simulink library "lfc"  (Simulink 8.2)
settings: Solver=ode1  StartTime=0.0  StopTime=Inf  FixedStep=0.001  RelTol=1e-3
PostLoadFcn:
  | , if any(exist('dsrtsu_mdlpostloadfcn', 'file') == [2, 3, 6]), try dsrtsu_mdlpostloadfcn('Execute', bdroot); catch fprintf('Error in PostLoadFcn (dsrtsu_mdlpostloadfcn) for model "%s":\n %s\n', bdroot, lasterr); end, end,
undefined symbols (not defined in the file or in its folder): ALFC_CenterC0_m, ALFC_ErrorY_m, ALFC_VehSpd_X_kph, C_TASK_5MS_S, C_TICK_TIME_S, ENUM_LFCSTATE_ADASFAILURE, ENUM_LFCSTATE_AUTOSTEERING, ENUM_LFCSTATE_DEGRADED, ENUM_LFCSTATE_DISABLED, ENUM_LFCSTATE_EPSRECOVERYPENDING, ENUM_LFCSTATE_OFF, ENUM_LFCSTATE_SOFTEN, ENUM_LFCSTATE_STANDBY, FALSE, KAPP_StrCenterOffset_deg, KAPP_Wheel2SteerRatio_rat, KAPP_WheelBase_m, KLFC_DDecRate_m, KLFC_DIncRate_m, KLFC_IGainLowerLimit_rad, KLFC_IGainUpperLimit_rad, MLFC_C0ErrorDist_m, MLFC_ControlGain_rat, MLFC_KgainRatio_rat, MLFC_KusCoeff_rat, MLFC_LookAheadDistGain_rat, TRUE
libraries: hcu_lib x7, simulink x2
settings Model: DSRTSU_INTERNAL_RTI_VER=450  DSRTSU_INTERNAL_RTI_TYPE=rti1401  RTICANMMDATA=struct('GeneralSetupData',struct('modelroot','C:\ADAS\trunk\ADAS_Softwares\HTDragon\software\sw_development\arch\app\lfc','generalsettings',struct('filesettings',struct('destfolder',struct('Name','RTICANMM_FILES','Check',1),'buildfolder',struct('Name','.','Check',1),'AbsDestfolder',struct('Name','C:\ADAS\trunk\ADAS_Softwares\HTDragon\software\sw_development\arch\app\lfc\RTICANMM_FILES'),'AbsBuildfolder',struct('Name','C:\ADAS\trunk\ADAS_Softwares\HTDragon\software\sw_development\arch\app\lfc'))),'options',struct('addpaths',1,'rmpaths',1,'addtrcexclusion',logical(1),'cannavigator',struct('checkmonitoring',0),'show_usrtrc',0,'use_usrtrc',0),'advanced',struct('options',[1 1 1 1 1 1 1 1 1 1 1 1 1 1 1 1 1 1 1 1 1 1 1 1 1 1 1 1 1 1 1 1 1 1 1 1 1 1 1 1 1 1 1 1 1 1 1 1 1 1 1 1 1 1 1 1 1 1 1 1 1 1 1 1 1 1 1 1 1 1 1 1 1 1 1 1 1 1 1 1 1 1 1 1 1 1 1 1 1 1 1 1 1 1 1 1 1 1 1 1]),'MPSetup',{{}},'modelname','lfc','block','lfc'))  DSRTSU_INTERNAL_RTIFPGA=40  Creator=14014  LastModifiedBy=13192

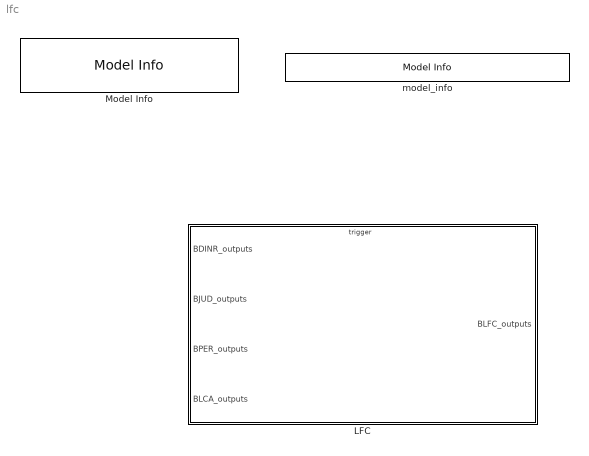
== system lfc ==
  LFC : Subsystem
  Model Info : simulink/Model-Wide Utilities/Model Info  InitialBlockCM=None  BlockCM=None  Frame=on  DisplayStringWithTags=|  HorizontalTextAlignment=Left  LeftAlignmentValue=0.02  SourceBlockDiagram=lfc  TagMaxNumber=20
      | Model Version        : %<ModelVersion>
      | Creator                   : %<Creator>
      | Last Modified by    : %<LastModifiedBy>
  model_info : simulink/Model-Wide Utilities/Model Info  InitialBlockCM=None  BlockCM=None  Frame=on  DisplayStringWithTags=$Id: lfc.mdl 1621 2017-09-19 03:18:21Z bcluan $  HorizontalTextAlignment=Center  LeftAlignmentValue=0.5  SourceBlockDiagram=lfc  TagMaxNumber=20

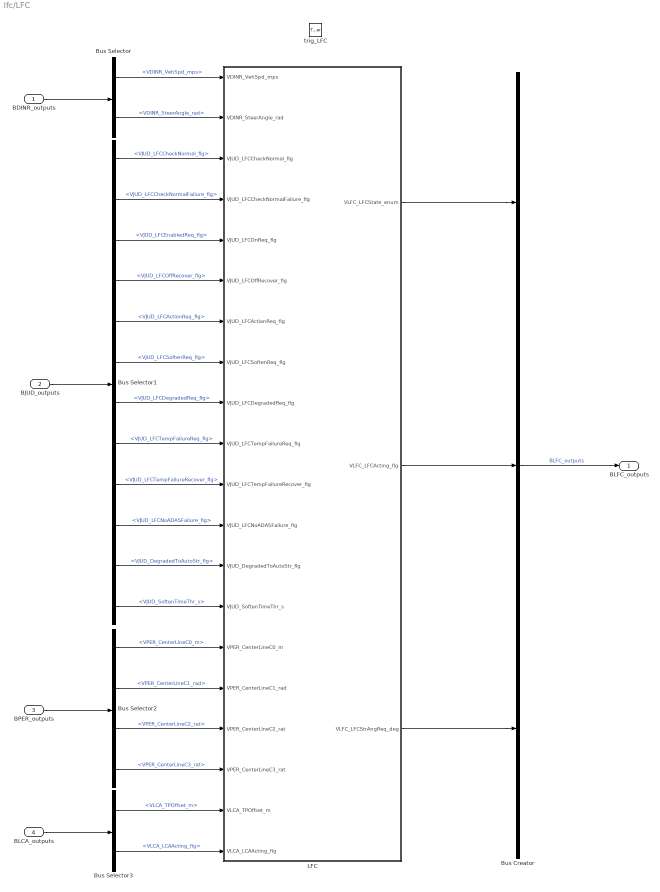
== system lfc/LFC ==
  BDINR_outputs : Inport  OutDataTypeStr=Bus: BDINR_outputs
  BJUD_outputs : Inport  Port=2  OutDataTypeStr=Bus: BJUD_outputs
  BPER_outputs : Inport  Port=3  OutDataTypeStr=Bus: BPER_outputs
  BLCA_outputs : Inport  Port=4  OutDataTypeStr=Bus: BLCA_outputs
  trig_LFC : TriggerPort  TriggerType=function-call
      settings: AttributesFormatString=State = %<StatesWhenEnabling>
  Bus Creator : BusCreator  Inputs=3  OutDataTypeStr=Bus: BLFC_outputs
  Bus Selector : BusSelector  OutputSignals=VDINR_VehSpd_mps,VDINR_SteerAngle_rad
  Bus Selector1 : BusSelector  OutputSignals=VJUD_LFCCheckNormal_flg,VJUD_LFCCheckNormalFailure_flg,VJUD_LFCEnabledReq_flg,VJUD_LFCOffRecover_flg,VJUD_LFCActionReq_flg,VJUD_LFCSoftenReq_flg,VJUD_LFCDegradedReq_flg,VJUD_LFCTempFailureReq_flg,VJUD_LFCTempFailureRecover_flg,VJUD_LFCNoADASFailure_flg,VJUD_DegradedToAutoStr_flg,VJUD_SoftenTimeThr_s
  Bus Selector2 : BusSelector  OutputSignals=VPER_CenterLineC0_m,VPER_CenterLineC1_rad,VPER_CenterLineC2_rat,VPER_CenterLineC3_rat
  Bus Selector3 : BusSelector  OutputSignals=VLCA_TPOffset_m,VLCA_LCAActing_flg
  LFC : Subsystem
  BLFC_outputs : Outport  OutDataTypeStr=Bus: BLFC_outputs
  wires:
  Bus Creator/1 -> BLFC_outputs/1  "BLFC_outputs"
  BDINR_outputs/1 -> Bus Selector/1
  BPER_outputs/1 -> Bus Selector2/1
  LFC/3(VLFC_LFCStrAngReq_deg) -> Bus Creator/3
  LFC/2(VLFC_LFCActing_flg) -> Bus Creator/2
  LFC/1(VLFC_LFCState_enum) -> Bus Creator/1
  BJUD_outputs/1 -> Bus Selector1/1
  Bus Selector/1 -> LFC/1(VDINR_VehSpd_mps)  "<VDINR_VehSpd_mps>"
  Bus Selector/2 -> LFC/2(VDINR_SteerAngle_rad)  "<VDINR_SteerAngle_rad>"
  Bus Selector1/1 -> LFC/3(VJUD_LFCCheckNormal_flg)  "<VJUD_LFCCheckNormal_flg>"
  Bus Selector1/3 -> LFC/5(VJUD_LFCOnReq_flg)  "<VJUD_LFCEnabledReq_flg>"
  Bus Selector1/4 -> LFC/6(VJUD_LFCOffRecover_flg)  "<VJUD_LFCOffRecover_flg>"
  Bus Selector1/5 -> LFC/7(VJUD_LFCActionReq_flg)  "<VJUD_LFCActionReq_flg>"
  Bus Selector1/6 -> LFC/8(VJUD_LFCSoftenReq_flg)  "<VJUD_LFCSoftenReq_flg>"
  Bus Selector1/7 -> LFC/9(VJUD_LFCDegradedReq_flg)  "<VJUD_LFCDegradedReq_flg>"
  Bus Selector1/8 -> LFC/10(VJUD_LFCTempFailureReq_flg)  "<VJUD_LFCTempFailureReq_flg>"
  Bus Selector1/9 -> LFC/11(VJUD_LFCTempFailureRecover_flg)  "<VJUD_LFCTempFailureRecover_flg>"
  Bus Selector1/10 -> LFC/12(VJUD_LFCNoADASFailure_flg)  "<VJUD_LFCNoADASFailure_flg>"
  Bus Selector1/11 -> LFC/13(VJUD_DegradedToAutoStr_flg)  "<VJUD_DegradedToAutoStr_flg>"
  BLCA_outputs/1 -> Bus Selector3/1
  Bus Selector1/12 -> LFC/14(VJUD_SoftenTimeThr_s)  "<VJUD_SoftenTimeThr_s>"
  Bus Selector2/4 -> LFC/18(VPER_CenterLineC3_rat)  "<VPER_CenterLineC3_rat>"
  Bus Selector2/2 -> LFC/16(VPER_CenterLineC1_rad)  "<VPER_CenterLineC1_rad>"
  Bus Selector2/1 -> LFC/15(VPER_CenterLineC0_m)  "<VPER_CenterLineC0_m>"
  Bus Selector2/3 -> LFC/17(VPER_CenterLineC2_rat)  "<VPER_CenterLineC2_rat>"
  Bus Selector3/1 -> LFC/19(VLCA_TPOffset_m)  "<VLCA_TPOffset_m>"
  Bus Selector3/2 -> LFC/20(VLCA_LCAActing_flg)  "<VLCA_LCAActing_flg>"
  Bus Selector1/2 -> LFC/4(VJUD_LFCCheckNormalFailure_flg)  "<VJUD_LFCCheckNormalFailure_flg>"

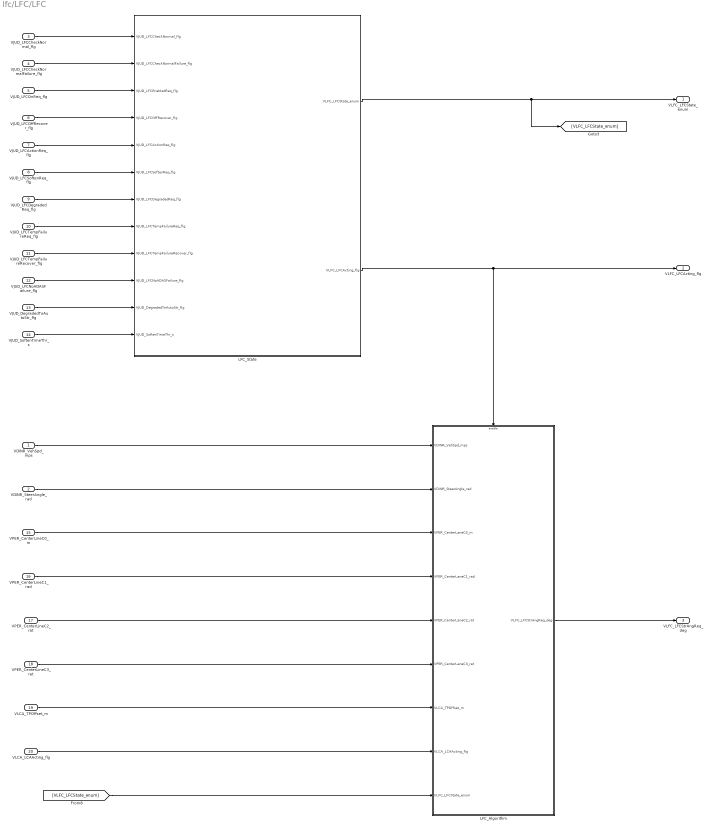
== system lfc/LFC/LFC ==
  VDINR_VehSpd_mps : Inport
  VDINR_SteerAngle_rad : Inport  Port=2
  VJUD_LFCCheckNormal_flg : Inport  Port=3
  VJUD_LFCCheckNormalFailure_flg : Inport  Port=4
  VJUD_LFCOnReq_flg : Inport  Port=5
  VJUD_LFCOffRecover_flg : Inport  Port=6
  VJUD_LFCActionReq_flg : Inport  Port=7
  VJUD_LFCSoftenReq_flg : Inport  Port=8
  VJUD_LFCDegradedReq_flg : Inport  Port=9
  VJUD_LFCTempFailureReq_flg : Inport  Port=10
  VJUD_LFCTempFailureRecover_flg : Inport  Port=11
  VJUD_LFCNoADASFailure_flg : Inport  Port=12
  VJUD_DegradedToAutoStr_flg : Inport  Port=13
  VJUD_SoftenTimeThr_s : Inport  Port=14
  VPER_CenterLineC0_m : Inport  Port=15
  VPER_CenterLineC1_rad : Inport  Port=16
  VPER_CenterLineC2_rat : Inport  Port=17
  VPER_CenterLineC3_rat : Inport  Port=18
  VLCA_TPOffset_m : Inport  Port=19
  VLCA_LCAActing_flg : Inport  Port=20
  LFC_Algorithm : Subsystem  TreatAsAtomicUnit=on
  LFC_State : Stateflow chart  TreatAsAtomicUnit=on
  VLFC_LFCState_enum : Outport  OutputWhenDisabled=reset  InitialOutput=[0]
  VLFC_LFCActing_flg : Outport  Port=2  OutputWhenDisabled=reset  InitialOutput=[0]
  VLFC_LFCStrAngReq_deg : Outport  Port=3  OutputWhenDisabled=reset  InitialOutput=[0]
  wires:
  [VLFC_LFCState_enum] -> LFC_Algorithm/9(VLFC_LFCState_enum)
  VLCA_LCAActing_flg/1 -> LFC_Algorithm/8(VLCA_LCAActing_flg)
  VLCA_TPOffset_m/1 -> LFC_Algorithm/7(VLCA_TPOffset_m)
  VJUD_DegradedToAutoStr_flg/1 -> LFC_State/11(VJUD_DegradedToAutoStr_flg)
  VJUD_LFCNoADASFailure_flg/1 -> LFC_State/10(VJUD_LFCNoADASFailure_flg)
  VJUD_LFCTempFailureRecover_flg/1 -> LFC_State/9(VJUD_LFCTempFailureRecover_flg)
  VJUD_LFCTempFailureReq_flg/1 -> LFC_State/8(VJUD_LFCTempFailureReq_flg)
  VJUD_SoftenTimeThr_s/1 -> LFC_State/12(VJUD_SoftenTimeThr_s)
  LFC_State/1(VLFC_LFCState_enum) -> VLFC_LFCState_enum/1, [VLFC_LFCState_enum]
  LFC_State/2(VLFC_LFCActing_flg) -> VLFC_LFCActing_flg/1, LFC_Algorithm/Enable
  VJUD_LFCDegradedReq_flg/1 -> LFC_State/7(VJUD_LFCDegradedReq_flg)
  VJUD_LFCSoftenReq_flg/1 -> LFC_State/6(VJUD_LFCSoftenReq_flg)
  VJUD_LFCActionReq_flg/1 -> LFC_State/5(VJUD_LFCActionReq_flg)
  VJUD_LFCOffRecover_flg/1 -> LFC_State/4(VJUD_LFCOffRecover_flg)
  VJUD_LFCOnReq_flg/1 -> LFC_State/3(VJUD_LFCEnabledReq_flg)
  VJUD_LFCCheckNormal_flg/1 -> LFC_State/1(VJUD_LFCCheckNormal_flg)
  LFC_Algorithm/1(VLFC_LFCStrAngReq_deg) -> VLFC_LFCStrAngReq_deg/1
  VDINR_SteerAngle_rad/1 -> LFC_Algorithm/2(VDINR_SteerAngle_rad)
  VDINR_VehSpd_mps/1 -> LFC_Algorithm/1(VDINR_VehSpd_mps)
  VPER_CenterLineC0_m/1 -> LFC_Algorithm/3(VPER_CenterLaneC0_m)
  VPER_CenterLineC1_rad/1 -> LFC_Algorithm/4(VPER_CenterLaneC1_rad)
  VPER_CenterLineC2_rat/1 -> LFC_Algorithm/5(VPER_CenterLaneC2_rat)
  VPER_CenterLineC3_rat/1 -> LFC_Algorithm/6(VPER_CenterLaneC3_rat)
  VJUD_LFCCheckNormalFailure_flg/1 -> LFC_State/2(VJUD_LFCCheckNormalFailure_flg)

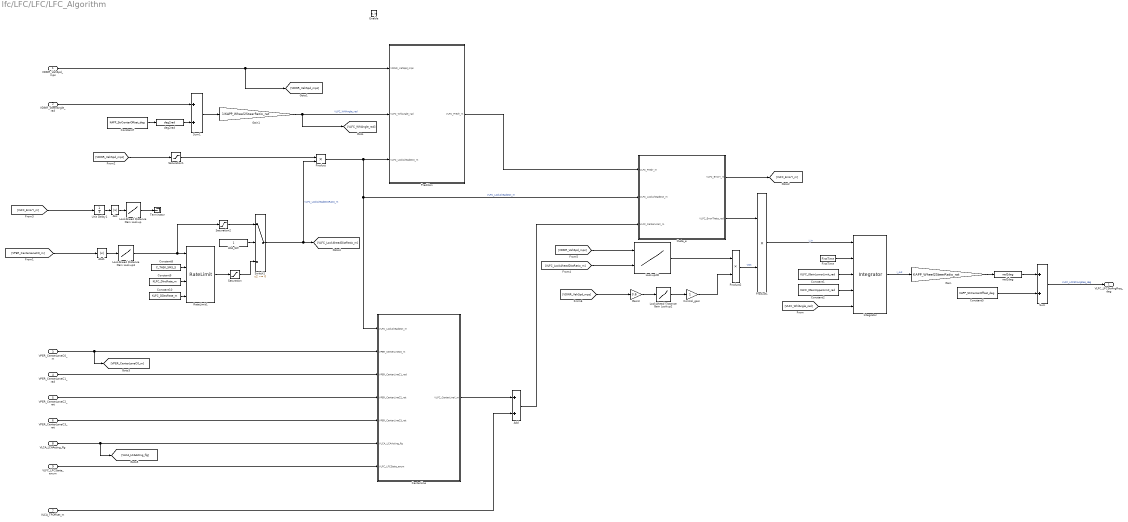
== system lfc/LFC/LFC/LFC_Algorithm ==
  VDINR_VehSpd_mps : Inport
  VDINR_SteerAngle_rad : Inport  Port=2
  VPER_CenterLaneC0_m : Inport  Port=3
  VPER_CenterLaneC1_rad : Inport  Port=4
  VPER_CenterLaneC2_rat : Inport  Port=5
  VPER_CenterLaneC3_rat : Inport  Port=6
  VLCA_TPOffset_m : Inport  Port=7
  VLCA_LCAActing_flg : Inport  Port=8
  VLFC_LFCState_enum : Inport  Port=9
  Enable : EnablePort  StatesWhenEnabling=reset
  Abs : Abs
  Abs1 : Abs
  Add : Sum
  CenterLine : Subsystem  TreatAsAtomicUnit=on
  Constant1 : Constant  Value=KLFC_IGainLowerLimit_rad
  Constant10 : Constant  Value=KLFC_DDecRate_m  OutDataTypeStr=single
  Constant2 : Constant  Value=KLFC_IGainUpperLimit_rad
  Constant5 : Constant  Value=KAPP_StrCenterOffset_deg
  Constant7 : Constant  Value=KAPP_StrCenterOffset_deg
  Constant8 : Constant  Value=C_TASK_5MS_S  OutDataTypeStr=single
  Constant9 : Constant  Value=KLFC_DIncRate_m  OutDataTypeStr=single
  Control_gain : Gain
  FirstTime : hcu_lib/FirstTime
  Gain : Gain  Gain=KAPP_Wheel2SteerRatio_rat
  Gain1 : Gain  Gain=1/KAPP_Wheel2SteerRatio_rat
  Gain3 : Gain  Gain=3.6
  Integrator : hcu_lib/Integrator  SystemSampleTime=-1
  LDA_SW : Constant  OutDataTypeStr=boolean
  LookAhead Distance Gain Lookup : Lookup  InputValues=ALFC_ErrorY_m  Table=MLFC_LookAheadDistGain_rat  LookUpMeth=Interpolation-Use End Values
      settings: AttributesFormatString=%<InputValues>\n%<Table>
  LookAhead Distance Gain Lookup2 : Lookup  InputValues=ALFC_VehSpd_X_kph  Table=MLFC_KgainRatio_rat  LookUpMeth=Interpolation-Use End Values
      settings: AttributesFormatString=%<InputValues>\n%<Table>
  LookAhead Distance Gain Lookup3 : Lookup  InputValues=ALFC_CenterC0_m  Table=MLFC_C0ErrorDist_m  LookUpMeth=Interpolation-Use End Values
      settings: AttributesFormatString=%<InputValues>\n%<Table>
  Lookup2D : Lookup2D  RowIndex=ALFC_VehSpd_X_mps  ColumnIndex=ALFC_LookAheadDist_Y_m  Table=MLFC_ControlGain_rat  LookUpMeth=Interpolation-Use End Values  OutDataTypeStr=single
      settings: AttributesFormatString=|
      | <row=%<RowIndex>>
      | <column=%<ColumnIndex>>
      | <table=%<Table>>
  Predition : Subsystem  TreatAsAtomicUnit=on
  Product : Product  RndMeth=Zero
  Product1 : Product  RndMeth=Zero
  Product2 : Product  RndMeth=Zero
  RateLimit1 : hcu_lib/RateLimit  SystemSampleTime=-1
  Saturation : Saturate  UpperLimit=2  LowerLimit=1
      settings: AttributesFormatString=upper = %<UpperLimit>\nlower = %<LowerLimit>
  Saturation1 : Saturate  UpperLimit=41.66  LowerLimit=2.78
      settings: AttributesFormatString=upper = %<UpperLimit>\nlower = %<LowerLimit>
  Saturation2 : Saturate  UpperLimit=2  LowerLimit=1.5
      settings: AttributesFormatString=upper = %<UpperLimit>\nlower = %<LowerLimit>
  Sum : Sum
  Sum1 : Sum
  Switch1 : Switch  Criteria=u2 ~= 0
      settings: AttributesFormatString=%<Criteria>
  Terminator : Terminator
  Unit Delay1 : UnitDelay  SampleTime=-1
  deg2rad : hcu_lib/deg2rad
  rad2deg : hcu_lib/rad2deg
  theta_e : Subsystem  TreatAsAtomicUnit=on
  VLFC_LFCStrAngReq_deg : Outport  OutputWhenDisabled=reset  InitialOutput=[0]
  wires:
  VLFC_LFCState_enum/1 -> CenterLine/7(VLFC_LFCState_enum)
  Control_gain/1 -> Product2/2
  Product1/1 -> Integrator/1  "I_in"
  Product2/1 -> Product1/2  "VDK"
  theta_e/2(VLFC_ErrorTheta_rad) -> Product1/1
  VLCA_LCAActing_flg/1 -> [VLCA_LCAActing_flg], CenterLine/6(VLCA_LCAActing_flg)
  Constant2/1 -> Integrator/4
  Constant1/1 -> Integrator/3
  rad2deg/1 -> Sum/1
  Predition/1(VLFC_PredY_m) -> theta_e/1(VLFC_PredY_m)
  [VLFC_WhlAngle_rad] -> Integrator/5
  VDINR_SteerAngle_rad/1 -> Sum1/1
  Gain/1 -> rad2deg/1
  theta_e/1(VLFC_ErrorY_m) -> [VLFC_ErrorY_m]
  VDINR_VehSpd_mps/1 -> [VDINR_VehSpd_mps], Predition/1(VDINR_VehSpd_mps)
  Gain1/1 -> [VLFC_WhlAngle_rad], Predition/2(VLFC_WhlAngle_rad)  "VLFC_WhlAngle_rad"
  FirstTime/1 -> Integrator/2
  Constant5/1 -> Sum/2
  Sum/1 -> VLFC_LFCStrAngReq_deg/1  "VLFC_LFCStrAngReq_deg"
  Integrator/1 -> Gain/1  "I_out"
  Constant7/1 -> deg2rad/1
  deg2rad/1 -> Sum1/2
  Sum1/1 -> Gain1/1
  VPER_CenterLaneC0_m/1 -> [VPER_CenterLaneC0_m], CenterLine/2(VPER_CenterLineC0_m)
  VPER_CenterLaneC1_rad/1 -> CenterLine/3(VPER_CenterLineC1_rad)
  VPER_CenterLaneC2_rat/1 -> CenterLine/4(VPER_CenterLineC2_rat)
  VPER_CenterLaneC3_rat/1 -> CenterLine/5(VPER_CenterLineC3_rat)
  [VDINR_VehSpd_mps] -> Saturation1/1
  [VLFC_ErrorY_m] -> Unit Delay1/1
  Unit Delay1/1 -> Abs/1
  Abs/1 -> LookAhead Distance Gain Lookup/1
  [VDINR_VehSpd_mps] -> Lookup2D/1
  [VLFC_LookAheadDistRatio_m] -> Lookup2D/2
  Constant9/1 -> RateLimit1/3
  Constant8/1 -> RateLimit1/2
  RateLimit1/1 -> Saturation/1
  [VPER_CenterLaneC0_m] -> Abs1/1
  Abs1/1 -> LookAhead Distance Gain Lookup3/1
  Product/1 -> CenterLine/1(VLFC_LookAheadDist_m), theta_e/2(VLFC_LookAheadDist_m), Predition/3(VLFC_LookAheadDist_m)  "VLFC_LookAheadDist_m"
  LookAhead Distance Gain Lookup/1 -> Terminator/1
  LookAhead Distance Gain Lookup3/1 -> Saturation2/1, RateLimit1/1
  [VDINR_VehSpd_mps] -> Gain3/1
  Gain3/1 -> LookAhead Distance Gain Lookup2/1
  Saturation1/1 -> Product/1
  Lookup2D/1 -> Product2/1
  LookAhead Distance Gain Lookup2/1 -> Control_gain/1
  Constant10/1 -> RateLimit1/4
  CenterLine/1(VLFC_CenterLineY_m) -> Add/1
  Saturation2/1 -> Switch1/1
  Saturation/1 -> Switch1/3
  Switch1/1 -> Product/2, [VLFC_LookAheadDistRatio_m]  "VLFC_LookAheadDistRatio_m"
  LDA_SW/1 -> Switch1/2
  Add/1 -> theta_e/3(VLFC_CenterLineY_m)
  VLCA_TPOffset_m/1 -> Add/2

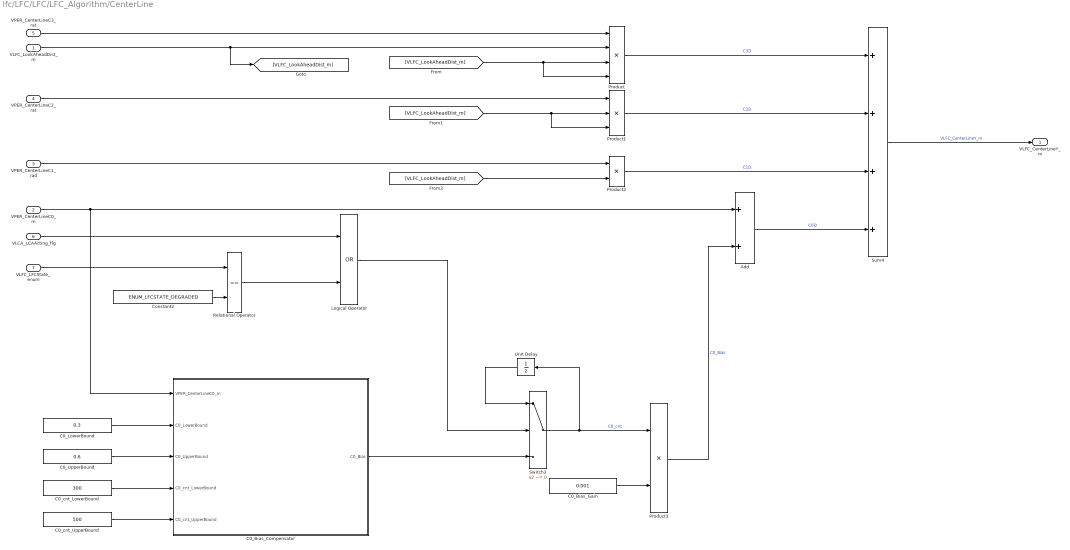
== system lfc/LFC/LFC/LFC_Algorithm/CenterLine ==
  VLFC_LookAheadDist_m : Inport
  VPER_CenterLineC0_m : Inport  Port=2
  VPER_CenterLineC1_rad : Inport  Port=3
  VPER_CenterLineC2_rat : Inport  Port=4
  VPER_CenterLineC3_rat : Inport  Port=5
  VLCA_LCAActing_flg : Inport  Port=6
  VLFC_LFCState_enum : Inport  Port=7
  Add : Sum
  C0_Bias_Compensator : Stateflow chart  TreatAsAtomicUnit=on
  C0_Bias_Gain : Constant  Value=0.001  OutDataTypeStr=single
  C0_LowerBound : Constant  Value=0.3  OutDataTypeStr=single
  C0_UpperBound : Constant  Value=0.6  OutDataTypeStr=single
  C0_cnt_LowerBound : Constant  Value=300  OutDataTypeStr=single
  C0_cnt_UpperBound : Constant  Value=500  OutDataTypeStr=single
  Constant2 : Constant  Value=ENUM_LFCSTATE_DEGRADED
  Logical Operator : Logic  Operator=OR  AllPortsSameDT=off  OutDataTypeStr=boolean
  Product : Product  Inputs=4  RndMeth=Zero
  Product1 : Product  Inputs=3  RndMeth=Zero
  Product2 : Product  RndMeth=Zero
  Product3 : Product
  Relational Operator : RelationalOperator  Operator===  OutDataTypeStr=boolean
  Sum4 : Sum  Inputs=++++
  Switch3 : Switch  Criteria=u2 ~= 0
  Unit Delay : UnitDelay  SampleTime=-1
  VLFC_CenterLineY_m : Outport
  wires:
  [VLFC_LookAheadDist_m] -> Product2/2
  [VLFC_LookAheadDist_m] -> Product1/2, Product1/3
  [VLFC_LookAheadDist_m] -> Product/3, Product/4
  Unit Delay/1 -> Switch3/1
  Switch3/1 -> Product3/1, Unit Delay/1  "C0_cnt"
  C0_Bias_Compensator/1(C0_Bias) -> Switch3/3
  Logical Operator/1 -> Switch3/2
  Relational Operator/1 -> Logical Operator/2
  Constant2/1 -> Relational Operator/2
  VLFC_LFCState_enum/1 -> Relational Operator/1
  VLCA_LCAActing_flg/1 -> Logical Operator/1
  C0_cnt_UpperBound/1 -> C0_Bias_Compensator/5(C0_cnt_UpperBound)
  Product3/1 -> Add/2  "C0_Bias"
  Add/1 -> Sum4/4  "C0D"
  C0_Bias_Gain/1 -> Product3/2
  C0_cnt_LowerBound/1 -> C0_Bias_Compensator/4(C0_cnt_LowerBound)
  C0_UpperBound/1 -> C0_Bias_Compensator/3(C0_UpperBound)
  C0_LowerBound/1 -> C0_Bias_Compensator/2(C0_LowerBound)
  VPER_CenterLineC0_m/1 -> C0_Bias_Compensator/1(VPER_CenterLineC0_m), Add/1
  Product2/1 -> Sum4/3  "C1D"
  Product1/1 -> Sum4/2  "C2D"
  Product/1 -> Sum4/1  "C3D"
  VPER_CenterLineC1_rad/1 -> Product2/1
  VPER_CenterLineC2_rat/1 -> Product1/1
  VPER_CenterLineC3_rat/1 -> Product/1
  VLFC_LookAheadDist_m/1 -> Product/2, [VLFC_LookAheadDist_m]
  Sum4/1 -> VLFC_CenterLineY_m/1  "VLFC_CenterLineY_m"

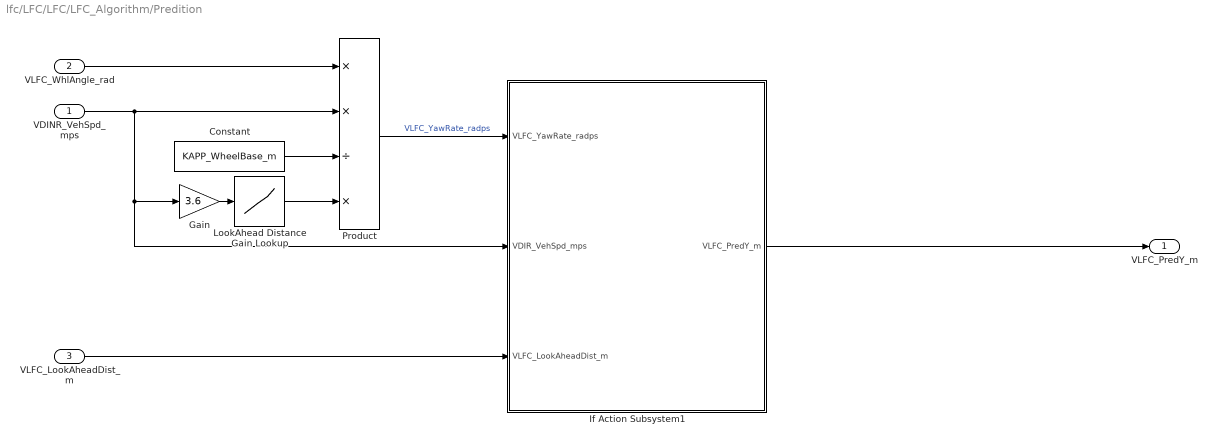
== system lfc/LFC/LFC/LFC_Algorithm/Predition ==
  VDINR_VehSpd_mps : Inport
  VLFC_WhlAngle_rad : Inport  Port=2
  VLFC_LookAheadDist_m : Inport  Port=3
  Constant : Constant  Value=KAPP_WheelBase_m
  Gain : Gain  Gain=3.6  ParamDataTypeStr=single
  If Action Subsystem1 : Subsystem  TreatAsAtomicUnit=on
  LookAhead Distance Gain Lookup : Lookup  InputValues=ALFC_VehSpd_X_kph  Table=MLFC_KusCoeff_rat  LookUpMeth=Interpolation-Use End Values
      settings: AttributesFormatString=%<InputValues>\n%<Table>
  Product : Product  Inputs=**/*  RndMeth=Zero
  VLFC_PredY_m : Outport
  wires:
  If Action Subsystem1/1(VLFC_PredY_m) -> VLFC_PredY_m/1
  VLFC_LookAheadDist_m/1 -> If Action Subsystem1/3(VLFC_LookAheadDist_m)
  Constant/1 -> Product/3
  VDINR_VehSpd_mps/1 -> Product/2, If Action Subsystem1/2(VDIR_VehSpd_mps), Gain/1
  VLFC_WhlAngle_rad/1 -> Product/1
  Product/1 -> If Action Subsystem1/1(VLFC_YawRate_radps)  "VLFC_YawRate_radps"
  LookAhead Distance Gain Lookup/1 -> Product/4
  Gain/1 -> LookAhead Distance Gain Lookup/1

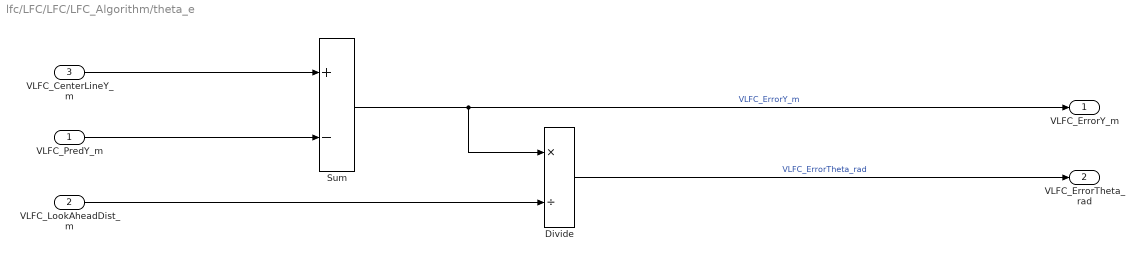
== system lfc/LFC/LFC/LFC_Algorithm/theta_e ==
  VLFC_PredY_m : Inport
  VLFC_LookAheadDist_m : Inport  Port=2
  VLFC_CenterLineY_m : Inport  Port=3
  Divide : Product  Inputs=*/
  Sum : Sum  Inputs=+-
  VLFC_ErrorY_m : Outport
  VLFC_ErrorTheta_rad : Outport  Port=2
  wires:
  Divide/1 -> VLFC_ErrorTheta_rad/1  "VLFC_ErrorTheta_rad"
  VLFC_LookAheadDist_m/1 -> Divide/2
  Sum/1 -> Divide/1, VLFC_ErrorY_m/1  "VLFC_ErrorY_m"
  VLFC_CenterLineY_m/1 -> Sum/1
  VLFC_PredY_m/1 -> Sum/2

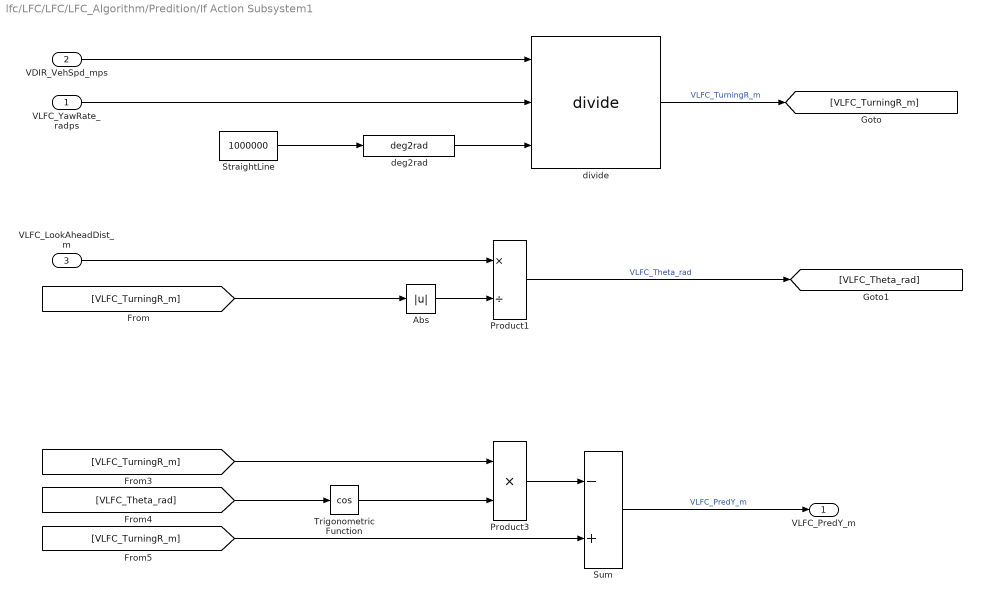
== system lfc/LFC/LFC/LFC_Algorithm/Predition/If Action Subsystem1 ==
  VLFC_YawRate_radps : Inport
  VDIR_VehSpd_mps : Inport  Port=2
  VLFC_LookAheadDist_m : Inport  Port=3
  Abs : Abs
  Product1 : Product  Inputs=*/  RndMeth=Zero
  Product3 : Product  Inputs=**  RndMeth=Zero
  StraightLine : Constant  Value=1000000  OutDataTypeStr=single
  Sum : Sum  Inputs=-+
  Trigonometric Function : Trigonometry  Operator=cos
  deg2rad : hcu_lib/deg2rad
  divide : hcu_lib/divide
  VLFC_PredY_m : Outport
  wires:
  deg2rad/1 -> divide/3
  StraightLine/1 -> deg2rad/1
  Trigonometric Function/1 -> Product3/2
  Sum/1 -> VLFC_PredY_m/1  "VLFC_PredY_m"
  [VLFC_TurningR_m] -> Sum/2
  Product3/1 -> Sum/1
  [VLFC_Theta_rad] -> Trigonometric Function/1
  [VLFC_TurningR_m] -> Product3/1
  Product1/1 -> [VLFC_Theta_rad]  "VLFC_Theta_rad"
  [VLFC_TurningR_m] -> Abs/1
  divide/1 -> [VLFC_TurningR_m]  "VLFC_TurningR_m"
  VLFC_LookAheadDist_m/1 -> Product1/1
  VLFC_YawRate_radps/1 -> divide/2
  VDIR_VehSpd_mps/1 -> divide/1
  Abs/1 -> Product1/2

== stateflow chart LFC/LFC/LFC_Algorithm/CenterLine/C0_Bias_Compensator ==
  (default) -> (junction 10)
  (junction 10) -> (junction 11) [order 1] : [VPER_CenterLineC0_m > C0_LowerBound]
  (junction 10) -> (junction 12) [order 2]
  (junction 11) -> (junction 14) : {C0_cnt= C0_cnt +1;
      | C0_Bias = C0_cnt;}
  (junction 12) -> (junction 13) [order 1] : [VPER_CenterLineC0_m < -C0_LowerBound]
  (junction 12) -> (junction 20) [order 2]
  (junction 13) -> (junction 22) : {C0_cnt = C0_cnt -1;
      | C0_Bias = C0_cnt;}
  (junction 14) -> (junction 15) [order 1] : [VPER_CenterLineC0_m > C0_UpperBound]
  (junction 14) -> (junction 16) [order 2]
  (junction 15) -> (junction 18) : {C0_cnt = C0_cnt +1;}
  (junction 16) -> (junction 17) [order 1] : [C0_cnt >= C0_cnt_UpperBound]
  (junction 18) -> (junction 19) [order 1] : [C0_cnt < 0]
  (junction 16) -> (junction 53) [order 2] : {C0_Bias = C0_cnt;}
  (junction 17) -> (junction 54) : {C0_cnt = C0_cnt_UpperBound;
      | C0_Bias = C0_cnt;}
  (junction 18) -> (junction 32) [order 2]
  (junction 19) -> (junction 30) : {C0_cnt = C0_cnt +2;}
  (junction 20) -> (junction 21) [order 1] : [C0_cnt <= -C0_cnt_UpperBound]
  (junction 22) -> (junction 23) [order 1] : [VPER_CenterLineC0_m < -C0_UpperBound]
  (junction 20) -> (junction 24) [order 2] : {C0_Bias = C0_cnt;}
  (junction 21) -> (junction 25) : {C0_cnt = -C0_cnt_UpperBound;
      | C0_Bias = C0_cnt}
  (junction 22) -> (junction 26) [order 2]
  (junction 23) -> (junction 28) : {C0_cnt = C0_cnt -1;}
  (junction 25) -> (junction 24)
  (junction 24) -> (junction 38)
  (junction 26) -> (junction 27) [order 1] : [C0_cnt <= -C0_cnt_UpperBound]
  (junction 28) -> (junction 29) [order 1] : [C0_cnt > 0]
  (junction 26) -> (junction 50) [order 2] : {C0_Bias = C0_cnt;}
  (junction 27) -> (junction 51) : {C0_cnt = -C0_cnt_UpperBound;
      | C0_Bias = C0_cnt}
  (junction 28) -> (junction 42) [order 2]
  (junction 29) -> (junction 40) : {C0_cnt = C0_cnt -2;}
  (junction 30) -> (junction 31) [order 1] : [C0_cnt < -C0_cnt_LowerBound]
  (junction 30) -> (junction 34) [order 2]
  (junction 31) -> (junction 36) : {C0_cnt = C0_cnt +2;}
  (junction 32) -> (junction 33) [order 1] : [C0_cnt >= C0_cnt_UpperBound]
  (junction 34) -> (junction 35) [order 1] : [C0_cnt >= C0_cnt_UpperBound]
  (junction 32) -> (junction 55) [order 2] : {C0_Bias = C0_cnt;}
  (junction 33) -> (junction 57) : {C0_cnt = C0_cnt_UpperBound;
      | C0_Bias = C0_cnt;}
  (junction 34) -> (junction 62) [order 2] : {C0_Bias = C0_cnt;}
  (junction 35) -> (junction 63) : {C0_cnt = C0_cnt_UpperBound;
      | C0_Bias = C0_cnt;}
  (junction 36) -> (junction 37) [order 1] : [C0_cnt >= C0_cnt_UpperBound]
  (junction 38) -> (junction 39) [order 1] : [C0_cnt >= C0_cnt_UpperBound]
  (junction 36) -> (junction 64) [order 2] : {C0_Bias = C0_cnt;}
  (junction 37) -> (junction 65) : {C0_cnt = C0_cnt_UpperBound;
      | C0_Bias = C0_cnt;}
  (junction 38) -> (junction 48) [order 2] : {C0_Bias = C0_cnt;}
  (junction 39) -> (junction 49) : {C0_cnt = C0_cnt_UpperBound;
      | C0_Bias = C0_cnt;}
  (junction 40) -> (junction 41) [order 1] : [C0_cnt > C0_cnt_LowerBound]
  (junction 40) -> (junction 44) [order 2]
  (junction 41) -> (junction 46) : {C0_cnt= C0_cnt -2;}
  (junction 42) -> (junction 43) [order 1] : [C0_cnt <= -C0_cnt_UpperBound]
  (junction 44) -> (junction 45) [order 1] : [C0_cnt <= -C0_cnt_UpperBound]
  (junction 42) -> (junction 52) [order 2] : {C0_Bias = C0_cnt;}
  (junction 43) -> (junction 56) : {C0_cnt = -C0_cnt_UpperBound;
      | C0_Bias = C0_cnt}
  (junction 44) -> (junction 58) [order 2] : {C0_Bias = C0_cnt;}
  (junction 45) -> (junction 59) : {C0_cnt = -C0_cnt_UpperBound;
      | C0_Bias= C0_cnt}
  (junction 46) -> (junction 47) [order 1] : [C0_cnt <= -C0_cnt_UpperBound]
  (junction 46) -> (junction 60) [order 2] : {C0_Bias = C0_cnt;}
  (junction 47) -> (junction 61) : {C0_cnt = -C0_cnt_UpperBound;
      | C0_Bias = C0_cnt}
  (junction 49) -> (junction 48)
  (junction 50) -> (junction 49)
  (junction 51) -> (junction 50)
  (junction 52) -> (junction 51)
  (junction 56) -> (junction 52)
  (junction 54) -> (junction 53)
  (junction 55) -> (junction 54)
  (junction 57) -> (junction 55)
  (junction 58) -> (junction 56)
  (junction 62) -> (junction 57)
  (junction 53) -> (junction 61)
  (junction 59) -> (junction 58)
  (junction 60) -> (junction 59)
  (junction 61) -> (junction 60)
  (junction 63) -> (junction 62)
  (junction 64) -> (junction 63)
  (junction 65) -> (junction 64)
  data: VPER_CenterLineC0_m input single; C0_LowerBound input single; C0_cnt local single; C0_Bias output single; C0_UpperBound input single; C0_cnt_LowerBound input single; C0_cnt_UpperBound input single

== stateflow chart LFC/LFC/LFC_State ==
  state NORMAL
    state ON
      state ENABLED
        state ACTIVE
          state ACTING
            state STEERING_CONTROL
              en:
              VLFC_LFCState_enum = ENUM_LFCSTATE_AUTOSTEERING;
              VLFC_LFCActing_flg = TRUE;
              VLFC_SoftenTimeLocal_s=0;
            state DEGRADED_CONTROL
              en:
              VLFC_LFCState_enum = ENUM_LFCSTATE_DEGRADED;
              VLFC_LFCActing_flg = TRUE;
              VLFC_SoftenTimeLocal_s=0;
            (default) -> STEERING_CONTROL
            STEERING_CONTROL -> DEGRADED_CONTROL : [VJUD_LFCDegradedReq_flg]
            DEGRADED_CONTROL -> STEERING_CONTROL : [VJUD_DegradedToAutoStr_flg]
          state SOFTEN
            en:
            VLFC_LFCState_enum = ENUM_LFCSTATE_SOFTEN;
            VLFC_LFCActing_flg = TRUE;
            VLFC_SoftenTimeLocal_s=0;
            du:
            VLFC_SoftenTimeLocal_s=VLFC_SoftenTimeLocal_s+C_TICK_TIME_S;
          (default) -> ACTING
          ACTING -> SOFTEN : [VJUD_LFCSoftenReq_flg]
        state STANDBY
          en:
          VLFC_LFCState_enum = ENUM_LFCSTATE_STANDBY;
          VLFC_LFCActing_flg = FALSE;
          VLFC_SoftenTimeLocal_s=0;
        (default) -> STANDBY
        STANDBY -> ACTIVE : [VJUD_LFCActionReq_flg]
      state OFF
        en:
        VLFC_LFCState_enum = ENUM_LFCSTATE_OFF;
        VLFC_LFCActing_flg = FALSE;
        VLFC_SoftenTimeLocal_s=0;
      (default) -> OFF
      OFF -> ENABLED : [VJUD_LFCEnabledReq_flg]
      ENABLED -> OFF : [VJUD_LFCOffRecover_flg ||...
          | VLFC_SoftenTimeLocal_s >= VJUD_SoftenTimeThr_s]
    state DISABLED
      en:
      VLFC_LFCState_enum = ENUM_LFCSTATE_DISABLED;
      VLFC_LFCActing_flg = FALSE;
      VLFC_SoftenTimeLocal_s=0;
    (default) -> DISABLED
    DISABLED -> ON : [VJUD_LFCCheckNormal_flg]
    ON -> DISABLED : [VJUD_LFCCheckNormalFailure_flg]
  state FAILURE_TEMPORARY
    state ADAS_FAILURE
      en:
      VLFC_LFCState_enum = ENUM_LFCSTATE_ADASFAILURE;
      VLFC_LFCActing_flg = FALSE;
      VLFC_SoftenTimeLocal_s=0;
    state EPS_RECOVERY_PENDING
      en:
      VLFC_LFCState_enum = ENUM_LFCSTATE_EPSRECOVERYPENDING;
      VLFC_LFCActing_flg = FALSE;
      VLFC_SoftenTimeLocal_s=0;
    (default) -> ADAS_FAILURE
    ADAS_FAILURE -> EPS_RECOVERY_PENDING : [VJUD_LFCNoADASFailure_flg]
    EPS_RECOVERY_PENDING -> ADAS_FAILURE : [!VJUD_LFCNoADASFailure_flg]
  (default) -> NORMAL
  NORMAL -> FAILURE_TEMPORARY : [VJUD_LFCTempFailureReq_flg]
  FAILURE_TEMPORARY -> NORMAL : [VJUD_LFCTempFailureRecover_flg]
  data: VLFC_LFCState_enum output double; VLFC_LFCActing_flg output double; VJUD_LFCCheckNormal_flg input double; VJUD_LFCCheckNormalFailure_flg input double; VJUD_LFCEnabledReq_flg input double; VJUD_LFCOffRecover_flg input double; VJUD_LFCActionReq_flg input double; VJUD_LFCSoftenReq_flg input double; VJUD_LFCDegradedReq_flg input double; VJUD_LFCTempFailureReq_flg input double; VJUD_LFCTempFailureRecover_flg input double; VJUD_LFCNoADASFailure_flg input double; TRUE parameter double; FALSE parameter double; VLFC_SoftenTimeLocal_s local single; ENUM_LFCSTATE_DISABLED parameter double; ENUM_LFCSTATE_OFF parameter double; ENUM_LFCSTATE_STANDBY parameter double; ENUM_LFCSTATE_AUTOSTEERING parameter double; ENUM_LFCSTATE_DEGRADED parameter double; ENUM_LFCSTATE_ADASFAILURE parameter double; ENUM_LFCSTATE_EPSRECOVERYPENDING parameter double; C_TICK_TIME_S parameter double; VJUD_DegradedToAutoStr_flg input double; VJUD_SoftenTimeThr_s input double; ENUM_LFCSTATE_SOFTEN parameter double
